simulink model "online_estimator_pe"  (R2019b)
settings: Solver=VariableStepAuto  StartTime=0.0  StopTime=500  RelTol=1e-3
values from neighbouring files (symbols this model uses):
  A = [-3  -4; 2  1]    [lin_state_estimator.mat]    (also in online_estimator.mat = [-0.25  3; -5  0])
  A_hat_init = [0  0; 0  0]    [online_estimator.mat]
  Am = [-2.5  30; -50  0]    [online_estimator.mat]
  b = 20    [directmrac workspace.mat]    (also in lin_state_estimator.mat = [1 0]; online_estimator.mat = [1 2.2])
  b_hat_init = [0 0]    [online_estimator.mat]
  Pm = [-0.32  -0.01; -0.01  -0.534166666667]    [online_estimator.mat]
  x_hat_init = [0 0]    [online_estimator.mat]
  x_init = [9 10]    [online_estimator.mat]
settings Model: Creator=chint  LastModifiedBy=chint

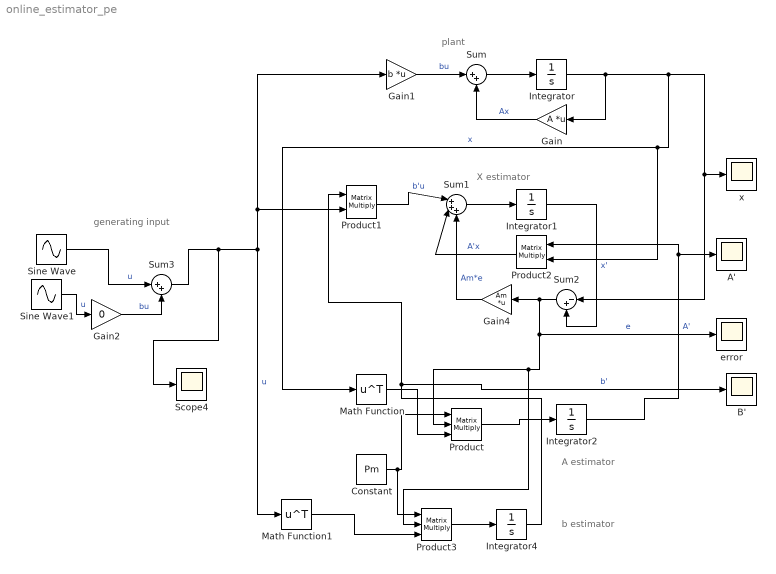
== system online_estimator_pe ==
  note: generating input
  note: plant
  note: X estimator
  note: A estimator
  note: b estimator
  A' : Scope
  B' : Scope
  Constant : Constant  Value=Pm
  Gain : Gain  Gain=A  Multiplication=Matrix(K*u)
  Gain1 : Gain  Gain=b  Multiplication=Matrix(K*u)
  Gain2 : Gain  Gain=0
  Gain4 : Gain  Gain=Am  Multiplication=Matrix(K*u)
  Integrator : Integrator  InitialCondition=x_init
  Integrator1 : Integrator  InitialCondition=x_hat_init
  Integrator2 : Integrator  InitialCondition=A_hat_init
  Integrator4 : Integrator  InitialCondition=b_hat_init
  Math Function : Math  Operator=transpose  SignedPower=off  SaturateOnIntegerOverflow=on
  Math Function1 : Math  Operator=transpose  SignedPower=off  SaturateOnIntegerOverflow=on
  Product : Product  Inputs=3  Multiplication=Matrix(*)
  Product1 : Product  Multiplication=Matrix(*)
  Product2 : Product  Multiplication=Matrix(*)
  Product3 : Product  Inputs=3  Multiplication=Matrix(*)
  Scope4 : Scope
  Sine Wave : Sin  Amplitude=10  Frequency=2  SampleTime=0
  Sine Wave1 : Sin  Amplitude=7  Frequency=3.6  Phase=pi/2  SampleTime=0
  Sum : Sum  Inputs=|++
  Sum1 : Sum  Inputs=|+++
  Sum2 : Sum  Inputs=|-+
  Sum3 : Sum  Inputs=|++
  error : Scope
  x : Scope
  wires:
  Integrator/1 -> Gain/1, x/1, Sum2/1, Product2/2, Math Function/1  "x"
  Sum/1 -> Integrator/1
  Gain/1 -> Sum/2  "Ax"
  Gain1/1 -> Sum/1  "bu"
  Product2/1 -> Sum1/2  "A'x"
  Product1/1 -> Sum1/1  "b'u"
  Integrator1/1 -> Sum2/2  "x'"
  Sum1/1 -> Integrator1/1
  Sum2/1 -> Product3/2, Product/2, error/1, Gain4/1  "e"
  Gain4/1 -> Sum1/3  "Am*e"
  Constant/1 -> Product3/1, Product/1
  Math Function/1 -> Product/3
  Product/1 -> Integrator2/1
  Integrator2/1 -> A'/1, Product2/1  "A'"
  Sum3/1 -> Scope4/1, Gain1/1, Product1/2, Math Function1/1  "u"
  Math Function1/1 -> Product3/3
  Product3/1 -> Integrator4/1
  Integrator4/1 -> Product1/1, B'/1  "b'"
  Sine Wave/1 -> Sum3/1  "u"
  Sine Wave1/1 -> Gain2/1  "u"
  Gain2/1 -> Sum3/2  "bu"
